simulink model "IP"  (R2025b)
settings: Solver=VariableStepAuto  StartTime=0.0  StopTime=10  RelTol=1e-3
PostLoadFcn:
  | rigid_body = importrobot('urdf\IP\urdf\IP.urdf');
  | rigid_body.DataFormat = 'column';
  | rigid_body.Gravity = [0 -9.81 0];
  | robot = get_robot_chain(rigid_body, 'rod','base_link');
  | robot.gravity = [0 -9.81 0];
  | m = 1;
  | M = 1;
  | l = 0.5;
  | g = 9.8;
  | A = [0, 0, 1, 0;
  |      0, 0, 0, 1;
  |      0, 3 * m * g / (4 * M + m), 0, 0;
  |      0, 6 * (M + m) * g / (l * (4 * M + m)), 0, 0];
  | B = [0;0;4/ (4 * M + m); 6 / (l * (4 * M + m))];
  | C = [1, 0, 0, 0];
  | D = 0;
  | init_pos = [0, 1e-4];
  | p = [-12, -10, -4 +  5.4575i, -4 -  5.4575i];
  | K = place(A, B, p);
libraries: aerolibanimutils x1
settings Model: Creator=Junch  LastModifiedBy=Junch

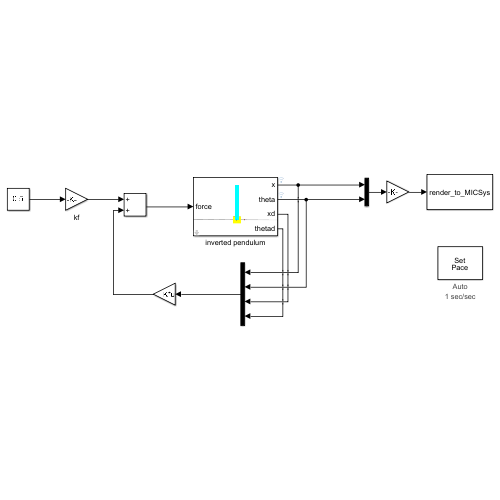
[thumbnail: Simulink's stored preview of the top-level diagram]
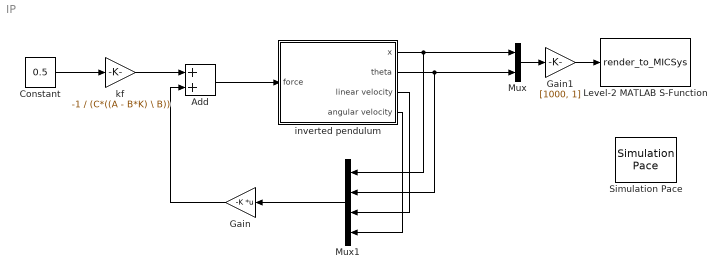
== system IP ==
  Add : Sum
  Constant : Constant  Value=0.5
  Gain : Gain  Gain=-K  Multiplication=Matrix(K*u)
  Gain1 : Gain  Gain=[1000, 1]
  Level-2 MATLAB S-Function : M-S-Function  FunctionName=render_to_MICSys
  Mux : Mux  Inputs=2
  Mux1 : Mux
  Simulation Pace : aerolibanimutils/Simulation Pace  SimulationPace=1  SleepMode=Auto  OutputPaceError=off  SampleTime=1/30
  inverted pendulum : Subsystem  mask{robot=robot, init_pos=[0, 0], Kd=[0, 0]}
      mask prompts: init_pos "intial position"; Kd "Kd (damping)"
      mask DialogControl ParameterGroupVar Prompt: 参数
      mask Display:
      | image('IP.png');
      | port_label('output', 1, 'x');
      | port_label('output', 2, 'theta');
      | port_label('output', 3, 'xd');
      | port_label('output', 4, 'thetad');
      | port_label('input', 1, 'force');
  kf : Gain  Gain=-1 / (C*((A - B*K) \ B))
  wires:
  Gain1/1 -> Level-2 MATLAB S-Function/1
  inverted pendulum/2(theta) -> Mux1/2, Mux/2
  Mux/1 -> Gain1/1
  Gain/1 -> Add/2
  inverted pendulum/1(x) -> Mux1/1, Mux/1
  inverted pendulum/3(linear velocity) -> Mux1/3
  inverted pendulum/4(angular velocity) -> Mux1/4
  Mux1/1 -> Gain/1
  Add/1 -> inverted pendulum/1(force)
  kf/1 -> Add/1
  Constant/1 -> kf/1

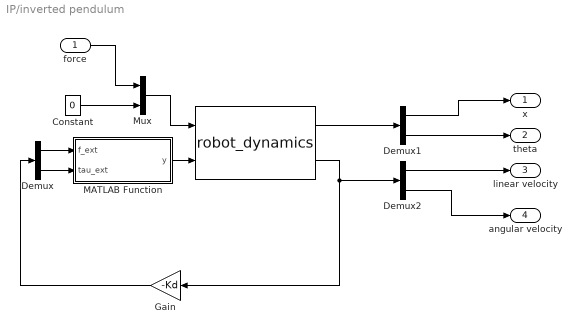
== system IP/inverted pendulum ==
  force : Inport
  " " : M-S-Function  FunctionName=robot_dynamics  Parameters=robot, init_pos, init_vel  mask{robot=robot, init_pos=init_pos, init_vel=zeros(1,2)}
      mask prompts: robot "robot struct:"; init_pos "init pos:"; init_vel "init velocity:"
      mask DialogControl ParameterGroupVar Prompt: 参数
      mask Display:
      | port_label('input', 1, 'control torque')
      | port_label('input', 2, 'external force')
      | port_label('output', 1, 'q')
      | port_label('output', 2, 'qd')
      | disp('Robot Dynamics');
  Constant : Constant  Value=0
  Demux : Demux  Outputs=2
  Demux1 : Demux  Outputs=2
  Demux2 : Demux  Outputs=2
  Gain : Gain  Gain=-Kd
  MATLAB Function : MATLAB Function  TreatAsAtomicUnit=on
  Mux : Mux  Inputs=2
  x : Outport
  theta : Outport  Port=2
  linear velocity : Outport  Port=3
  angular velocity : Outport  Port=4
  wires:
  Demux/1 -> MATLAB Function/1(f_ext)
  Constant/1 -> Mux/2
  force/1 -> Mux/1
  Gain/1 -> Demux/1
  Mux/1 -> " "/1
  MATLAB Function/1(y) -> " "/2
  " "/2 -> Demux2/1, Gain/1
  Demux/2 -> MATLAB Function/2(tau_ext)
  " "/1 -> Demux1/1
  Demux1/1 -> x/1
  Demux1/2 -> theta/1
  Demux2/1 -> linear velocity/1
  Demux2/2 -> angular velocity/1

== matlab function IP/inverted pendulum/MATLAB Function ==
  data: f_ext input; y output; tau_ext input
function y = fcn(f_ext, tau_ext)
%#codegen
y1 = [0, 0, 0, f_ext, 0, 0]';
y2 = [0, 0, tau_ext, 0, 0, 0]';
y = [y1, y2];
